simulink model "RC_Circuit_N18"  (R2020b)
settings: Solver=VariableStepAuto  StartTime=0.0  StopTime=1  RelTol=1e-3
model workspace (MAT data in the model file):
  Cp = 3.7334e-07
  Cs = 4.36284e-11
  L = 2.56583333333e-07
  R = 5.49453333333
libraries: powerlib x74
settings Model: OrderedModelArguments=off  Creator=zq001  LastModifiedBy=zq001
settings DebuggingCC: UnconnectedLineMsg=none

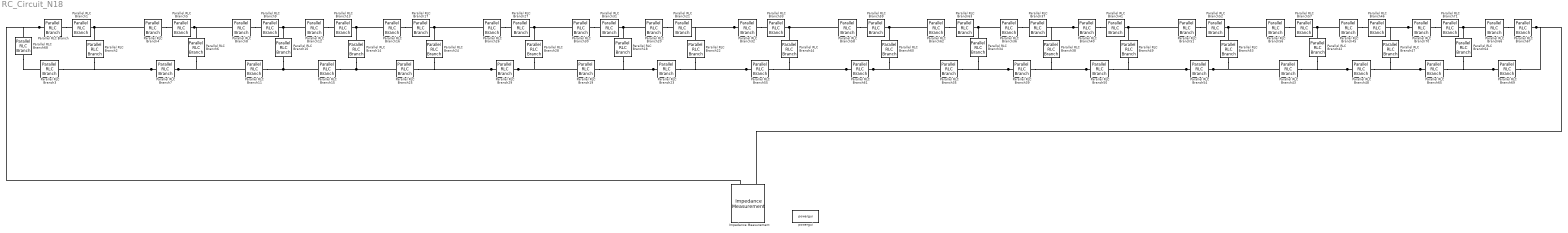
== system RC_Circuit_N18 ==
  Impedance Measurement : powerlib/Measurements/Impedance Measurement  LConnTagsString=+|-  Factor=1
      settings: SourceProductBaseCode=PS
  Parallel RLC Branch{,4,8,12,16,20,26,30,32,36,40,45,51,56,58,62,66,70} (18 alike) : powerlib/Elements/Parallel RLC Branch  LConnTagsString=a  RConnTagsString=__new0  BranchType=R  Resistance=R  Inductance=1e-3  SetiL0=off  InitialCurrent=0  Capacitance=1e-6  Setx0=off  InitialVoltage=0  Measurements=None
  Parallel RLC Branch{1,5,9,13,17,21,27,31,33,37,41,46,52,57,59,63,67,71} (18 alike) : powerlib/Elements/Parallel RLC Branch  LConnTagsString=a  RConnTagsString=__new0  BranchType=L  Resistance=1  Inductance=L  SetiL0=off  InitialCurrent=0  Capacitance=1e-6  Setx0=off  InitialVoltage=0  Measurements=None
  Parallel RLC Branch{2,6,10,14,18,22,24,28,34,38,42,44,47,49,53,60,64,68} (18 alike) : powerlib/Elements/Parallel RLC Branch  LConnTagsString=a  RConnTagsString=__new0  BranchType=C  Resistance=1  Inductance=1e-3  SetiL0=off  InitialCurrent=0  Capacitance=Cp  Setx0=off  InitialVoltage=0  Measurements=None
  Parallel RLC Branch{3,7,11,15,19,23,25,29,35,39,43,48,50,54..55,61,65,69} (18 alike) : powerlib/Elements/Parallel RLC Branch  LConnTagsString=a  RConnTagsString=__new0  BranchType=C  Resistance=1  Inductance=1e-3  SetiL0=off  InitialCurrent=0  Capacitance=Cs  Setx0=off  InitialVoltage=0  Measurements=None
  powergui : powerlib/powergui  Priority=1  SimulationMode=Continuous  SampleTime=50e-6  frequency=60  Iterations=50  frequencyindice=60  Pbase=100e6  ErrMax=1e-4  UnitsV=kV  UnitsW=MW  buscounter=0  FunctionMessages=off  echomessages=off  EnableUseOfTLC=off  CurrentSourceSwitches=off  DisableSnubberDevices=off  DisableRonSwitches=off  DisableVfSwitches=off  DisplayEquations=off  AutomaticDiscreteSolvers=off  SolverType=Tustin/Backward Euler (TBE)  Interpol=off  ExternalGateDelay=off  methode=off  Ts=100  x0status=blocks  SPID=on  SwTol=0  HookPort=off  NonlinearTolerance=1e-4  nMaxIteration=100  ContinueOnMaxIteration=off  RestoreLinks=warning  ResistiveCurrentMeasurement=off  Frange=[0:2:500]  Ylog=off  Xlog=off  ShowGrid=on  save=off  variable=ZData  structure=0  ZoomFFT=off  StartTime=0.0  cycles=1  DisplayStyle=1  fundamental=60  FreqAxis=off  MaxFrequency=1000  frequencyindicesteady=1  RmsSteady=1  display=off
  connections:
  Parallel RLC Branch1/RConn1 -- Parallel RLC Branch4/LConn1 -- Parallel RLC Branch2/LConn1
  Parallel RLC Branch10/RConn1 -- Parallel RLC Branch11/RConn1 -- Parallel RLC Branch15/LConn1
  Parallel RLC Branch71/RConn1 -- Parallel RLC Branch66/LConn1 -- Parallel RLC Branch64/LConn1
  Parallel RLC Branch33/RConn1 -- Parallel RLC Branch58/LConn1 -- Parallel RLC Branch44/LConn1
  Parallel RLC Branch31/RConn1 -- Parallel RLC Branch20/LConn1 -- Parallel RLC Branch18/LConn1
  Parallel RLC Branch/LConn1 -- Impedance Measurement/LConn1 -- Parallel RLC Branch68/LConn1
  Parallel RLC Branch14/RConn1 -- Parallel RLC Branch15/RConn1 -- Parallel RLC Branch25/LConn1
  Parallel RLC Branch69/LConn1 -- Parallel RLC Branch65/RConn1 -- Parallel RLC Branch64/RConn1
  Parallel RLC Branch5/RConn1 -- Parallel RLC Branch8/LConn1 -- Parallel RLC Branch6/LConn1
  Parallel RLC Branch61/LConn1 -- Parallel RLC Branch44/RConn1 -- Parallel RLC Branch55/RConn1
  Parallel RLC Branch52/RConn1 -- Parallel RLC Branch56/LConn1 -- Parallel RLC Branch53/LConn1
  Parallel RLC Branch67/RConn1 -- Impedance Measurement/LConn2 -- Parallel RLC Branch69/RConn1
  Parallel RLC Branch32/LConn1 -- Parallel RLC Branch21/RConn1 -- Parallel RLC Branch22/LConn1
  Parallel RLC Branch54/LConn1 -- Parallel RLC Branch49/RConn1 -- Parallel RLC Branch50/RConn1
  Parallel RLC Branch55/LConn1 -- Parallel RLC Branch23/RConn1 -- Parallel RLC Branch22/RConn1
  Parallel RLC Branch59/RConn1 -- Parallel RLC Branch62/LConn1 -- Parallel RLC Branch60/LConn1
  Parallel RLC Branch61/RConn1 -- Parallel RLC Branch35/LConn1 -- Parallel RLC Branch60/RConn1
  Parallel RLC Branch41/RConn1 -- Parallel RLC Branch51/LConn1 -- Parallel RLC Branch49/LConn1
  Parallel RLC Branch39/LConn1 -- Parallel RLC Branch35/RConn1 -- Parallel RLC Branch34/RConn1
  Parallel RLC Branch63/RConn1 -- Parallel RLC Branch36/LConn1 -- Parallel RLC Branch34/LConn1
  Parallel RLC Branch14/LConn1 -- Parallel RLC Branch13/RConn1 -- Parallel RLC Branch16/LConn1
  Parallel RLC Branch7/LConn1 -- Parallel RLC Branch2/RConn1 -- Parallel RLC Branch3/RConn1
  Parallel RLC Branch54/RConn1 -- Parallel RLC Branch43/LConn1 -- Parallel RLC Branch53/RConn1
  Parallel RLC Branch9/RConn1 -- Parallel RLC Branch12/LConn1 -- Parallel RLC Branch10/LConn1
  Parallel RLC Branch65/LConn1 -- Parallel RLC Branch48/RConn1 -- Parallel RLC Branch47/RConn1
  Parallel RLC Branch70/LConn1 -- Parallel RLC Branch46/RConn1 -- Parallel RLC Branch47/LConn1
  Parallel RLC Branch48/LConn1 -- Parallel RLC Branch43/RConn1 -- Parallel RLC Branch42/RConn1
  Parallel RLC Branch7/RConn1 -- Parallel RLC Branch11/LConn1 -- Parallel RLC Branch6/RConn1
  Parallel RLC Branch27/RConn1 -- Parallel RLC Branch30/LConn1 -- Parallel RLC Branch28/LConn1
  Parallel RLC Branch40/LConn1 -- Parallel RLC Branch37/RConn1 -- Parallel RLC Branch38/LConn1
  Parallel RLC Branch17/RConn1 -- Parallel RLC Branch26/LConn1 -- Parallel RLC Branch24/LConn1
  Parallel RLC Branch29/LConn1 -- Parallel RLC Branch24/RConn1 -- Parallel RLC Branch25/RConn1
  Parallel RLC Branch23/LConn1 -- Parallel RLC Branch19/RConn1 -- Parallel RLC Branch18/RConn1
  Parallel RLC Branch50/LConn1 -- Parallel RLC Branch39/RConn1 -- Parallel RLC Branch38/RConn1
  Parallel RLC Branch29/RConn1 -- Parallel RLC Branch19/LConn1 -- Parallel RLC Branch28/RConn1
  Parallel RLC Branch57/RConn1 -- Parallel RLC Branch45/LConn1 -- Parallel RLC Branch42/LConn1
  Parallel RLC Branch4/RConn1 -- Parallel RLC Branch5/LConn1
  Parallel RLC Branch51/RConn1 -- Parallel RLC Branch52/LConn1
  Parallel RLC Branch32/RConn1 -- Parallel RLC Branch33/LConn1
  Parallel RLC Branch36/RConn1 -- Parallel RLC Branch37/LConn1
  Parallel RLC Branch20/RConn1 -- Parallel RLC Branch21/LConn1
  Parallel RLC Branch70/RConn1 -- Parallel RLC Branch71/LConn1
  Parallel RLC Branch66/RConn1 -- Parallel RLC Branch67/LConn1
  Parallel RLC Branch8/RConn1 -- Parallel RLC Branch9/LConn1
  Parallel RLC Branch58/RConn1 -- Parallel RLC Branch59/LConn1
  Parallel RLC Branch/RConn1 -- Parallel RLC Branch1/LConn1
  Parallel RLC Branch68/RConn1 -- Parallel RLC Branch3/LConn1
  Parallel RLC Branch45/RConn1 -- Parallel RLC Branch46/LConn1
  Parallel RLC Branch12/RConn1 -- Parallel RLC Branch13/LConn1
  Parallel RLC Branch40/RConn1 -- Parallel RLC Branch41/LConn1
  Parallel RLC Branch30/RConn1 -- Parallel RLC Branch31/LConn1
  Parallel RLC Branch62/RConn1 -- Parallel RLC Branch63/LConn1
  Parallel RLC Branch26/RConn1 -- Parallel RLC Branch27/LConn1
  Parallel RLC Branch16/RConn1 -- Parallel RLC Branch17/LConn1
  Parallel RLC Branch56/RConn1 -- Parallel RLC Branch57/LConn1
